simulink model "GolfSwingZVCF"  (R2024b)
settings: Solver=VariableStepAuto  StartTime=0.0  StopTime=StopTime  MaxStep=0.001  RelTol=1e-3
PreLoadFcn:
  | cd(matlabdrive);
  | cd '2DModel';
PostLoadFcn:
  | %run SCRIPT_mdlWksGenerate.m;
  | mdlWks=get_param('GolfSwingZVCF','ModelWorkspace');
  | mdlWks.DataSource = 'MAT-File';
  | mdlWks.FileName = 'ModelInputs.mat';
  | mdlWks.reload;
model workspace: external: MAT-File ModelInputsZVCF.mat (data not in the file)
undefined symbols (not defined in the file): JointTorqueHip, JointTorqueLElbow, JointTorqueLScap, JointTorqueLShoulder, JointTorqueLWrist, JointTorqueRElbow, JointTorqueRScap, JointTorqueRShoulder, JointTorqueRWrist, JointTorqueTorso, X, Y, Z
libraries: nesl_utility x286, sm_lib x176, matrix_library x11, simulink_extras x2
(part 4 of 9)

== system GolfSwingZVCF/Club/ButtGlobal ==
  Buttx : nesl_utility/PS-Simulink Converter  PhysicalDomain=network_engine_domain  SubClassName=ps_output  LeftPortType=input  RightPortType=output  PseudoPeriodic=off  Frequencies=[]  VectorFormat=1-D array  Unit=inherit  AffineConversion=off
  Butty : nesl_utility/PS-Simulink Converter  PhysicalDomain=network_engine_domain  SubClassName=ps_output  LeftPortType=input  RightPortType=output  PseudoPeriodic=off  Frequencies=[]  VectorFormat=1-D array  Unit=inherit  AffineConversion=off
  Buttz : nesl_utility/PS-Simulink Converter  PhysicalDomain=network_engine_domain  SubClassName=ps_output  LeftPortType=input  RightPortType=output  PseudoPeriodic=off  Frequencies=[]  VectorFormat=1-D array  Unit=inherit  AffineConversion=off
  Transform Sensor : sm_lib/Frames and Transforms/Transform Sensor  MeasurementFrame=World  RotationSequence=XYX  SenseAngle=off  SenseAxis=off  SenseQ=off  SenseR=off  SenseRotationSequence=off  SenseOmegaX=off  SenseOmegaY=off  SenseOmegaZ=off  SenseOmega=off  SenseQDot=off  SenseRDot=off  SenseRotationSequenceDot=off  SenseAlphaX=off  SenseAlphaY=off  SenseAlphaZ=off  SenseAlpha=off  SenseQDDot=off  SenseRDDot=off  SenseX=on  SenseY=on  SenseZ=on  SenseXYZ=off  SenseRad=off  SenseAzim=off  SenseDist=off  SenseInc=off  SenseXDot=off  SenseYDot=off  SenseZDot=off  SenseXYZDot=off  SenseRadDot=off  SenseAzimDot=off  SenseDistDot=off  SenseIncDot=off  SenseXDDot=off  SenseYDDot=off  SenseZDDot=off  SenseXYZDDot=off  SenseRadDDot=off  SenseAzimDDot=off  SenseDistDDot=off  SenseIncDDot=off
  Conn1 : PMIOPort  Side=Right
  Conn2 : PMIOPort  Port=2  Side=Left
  connections:
  Buttx/LConn1 -- Transform Sensor/RConn2
  Buttz/LConn1 -- Transform Sensor/RConn4
  Butty/LConn1 -- Transform Sensor/RConn3
  Transform Sensor/LConn1 -- Conn2/RConn1
  Transform Sensor/RConn1 -- Conn1/RConn1

== system GolfSwingZVCF/Club/CHGlobal ==
  AoA Calculation : Subsystem
  CHS (m/s) : Subsystem
  CHSmph : Gain  Gain=2.23694
  CHvx : nesl_utility/PS-Simulink Converter  PhysicalDomain=network_engine_domain  SubClassName=ps_output  LeftPortType=input  RightPortType=output  PseudoPeriodic=off  Frequencies=[]  VectorFormat=1-D array  Unit=inherit  AffineConversion=off
  CHvy : nesl_utility/PS-Simulink Converter  PhysicalDomain=network_engine_domain  SubClassName=ps_output  LeftPortType=input  RightPortType=output  PseudoPeriodic=off  Frequencies=[]  VectorFormat=1-D array  Unit=inherit  AffineConversion=off
  CHvz : nesl_utility/PS-Simulink Converter  PhysicalDomain=network_engine_domain  SubClassName=ps_output  LeftPortType=input  RightPortType=output  PseudoPeriodic=off  Frequencies=[]  VectorFormat=1-D array  Unit=inherit  AffineConversion=off
  CHx : nesl_utility/PS-Simulink Converter  PhysicalDomain=network_engine_domain  SubClassName=ps_output  LeftPortType=input  RightPortType=output  PseudoPeriodic=off  Frequencies=[]  VectorFormat=1-D array  Unit=inherit  AffineConversion=off
  CHy : nesl_utility/PS-Simulink Converter  PhysicalDomain=network_engine_domain  SubClassName=ps_output  LeftPortType=input  RightPortType=output  PseudoPeriodic=off  Frequencies=[]  VectorFormat=1-D array  Unit=inherit  AffineConversion=off
  CHz : nesl_utility/PS-Simulink Converter  PhysicalDomain=network_engine_domain  SubClassName=ps_output  LeftPortType=input  RightPortType=output  PseudoPeriodic=off  Frequencies=[]  VectorFormat=1-D array  Unit=inherit  AffineConversion=off
  ClubheadPathUnitVector : Mux  Inputs=3
  Filtering Block : Subsystem  Commented=on
  Path Calculation : Subsystem
  Transform Sensor : sm_lib/Frames and Transforms/Transform Sensor  MeasurementFrame=World  RotationSequence=XYX  SenseAngle=off  SenseAxis=off  SenseQ=off  SenseR=off  SenseRotationSequence=off  SenseOmegaX=off  SenseOmegaY=off  SenseOmegaZ=off  SenseOmega=off  SenseQDot=off  SenseRDot=off  SenseRotationSequenceDot=off  SenseAlphaX=off  SenseAlphaY=off  SenseAlphaZ=off  SenseAlpha=off  SenseQDDot=off  SenseRDDot=off  SenseX=on  SenseY=on  SenseZ=on  SenseXYZ=off  SenseRad=off  SenseAzim=off  SenseDist=off  SenseInc=off  SenseXDot=on  SenseYDot=on  SenseZDot=on  SenseXYZDot=off  SenseRadDot=off  SenseAzimDot=off  SenseDistDot=off  SenseIncDot=off  SenseXDDot=off  SenseYDDot=off  SenseZDDot=off  SenseXYZDDot=off  SenseRadDDot=off  SenseAzimDDot=off  SenseDistDDot=off  SenseIncDDot=off
  UnitVectorX : Product  Inputs=*/
  UnitVectorY : Product  Inputs=*/
  UnitVectorZ : Product  Inputs=*/
  Clubhead : PMIOPort  Side=Right
  Global : PMIOPort  Port=2  Side=Left
  ClubPathUV : Outport
  CHSMPS : Outport  Port=2
  wires:
  CHvy/1 -> Path Calculation/1(Vy), AoA Calculation/2(Vy), UnitVectorY/1, CHS (m/s)/2(In2)  "CHvy"
  CHvx/1 -> AoA Calculation/1(Vx), Path Calculation/2(Vx), UnitVectorX/1, CHS (m/s)/1(In1)  "CHvx"
  CHvz/1 -> CHS (m/s)/3(In3), AoA Calculation/3(Vz), UnitVectorZ/1  "CHvz"
  UnitVectorZ/1 -> ClubheadPathUnitVector/3
  UnitVectorY/1 -> ClubheadPathUnitVector/2
  CHS (m/s)/1(ClubPathUV1) -> CHSMPS/1, CHSmph/1, UnitVectorZ/2, UnitVectorY/2, UnitVectorX/2  "CHSmpersec"
  UnitVectorX/1 -> ClubheadPathUnitVector/1
  ClubheadPathUnitVector/1 -> ClubPathUV/1  "ClubPathUV"
  CHSmph/1 -> Filtering Block/1(CHS (mph))  "CHS (mph)"
  connections:
  CHx/LConn1 -- Transform Sensor/RConn2
  CHz/LConn1 -- Transform Sensor/RConn4
  CHvz/LConn1 -- Transform Sensor/RConn7
  CHy/LConn1 -- Transform Sensor/RConn3
  Transform Sensor/RConn5 -- CHvx/LConn1
  CHvy/LConn1 -- Transform Sensor/RConn6
  Transform Sensor/LConn1 -- Global/RConn1
  Transform Sensor/RConn1 -- Clubhead/RConn1

== system GolfSwingZVCF/Club/Club COM Calculation ==
  Club COM : nesl_utility/PS-Simulink Converter  PhysicalDomain=network_engine_domain  SubClassName=ps_output  LeftPortType=input  RightPortType=output  PseudoPeriodic=off  Frequencies=[]  VectorFormat=1-D array  Unit=inherit  AffineConversion=off
  Club Mass : nesl_utility/PS-Simulink Converter  PhysicalDomain=network_engine_domain  SubClassName=ps_output  LeftPortType=input  RightPortType=output  PseudoPeriodic=off  Frequencies=[]  VectorFormat=1-D array  Unit=inherit  AffineConversion=off
  Inertia Sensor : sm_lib/Body Elements/Inertia Sensor  SensorExtent=BodyGroup  SpanWeldJoints=on  ExcludeGroundedBodies=off  MeasurementFrame=World  SenseMass=on  SenseCenterOfMass=on  SenseInertiaMatrix=off  SenseCenteredInertiaMatrix=off  SensePrincipalInertiaMatrix=off  SenseRotationMatrix=off  GraphicType=None  PrincipalInertiaFrameSize=20  GraphicVisPropType=SimpleVisualProperties  GraphicDiffuseColor=[0.5 0.5 0.5]  GraphicOpacity=1.0  GraphicSpecularColor=[0.5 0.5 0.5 1.0]  GraphicAmbientColor=[0.15 0.15 0.15 1.0]  GraphicEmissiveColor=[0.0 0.0 0.0 1.0]  GraphicShininess=75
  Club : PMIOPort  Side=Left
  ClubCOM : Outport
  wires:
  Club COM/1 -> ClubCOM/1  "ClubCOM"
  connections:
  Club COM/LConn1 -- Inertia Sensor/RConn2
  Inertia Sensor/LConn1 -- Club/RConn1
  Inertia Sensor/RConn1 -- Club Mass/LConn1

== system GolfSwingZVCF/Club/Clubhead Air Resistance Calculator ==
  CHSmps : Inport
  ClubPathUV : Inport  Port=2
  Add : Sum  Inputs=+++
  Air Resistance : sm_lib/Forces and Torques/External Force and Torque  EnableForceX=off  EnableForceY=off  EnableForceZ=off  EnableForce=on  ForceResolutionFrame=World  EnableTorqueX=off  EnableTorqueY=off  EnableTorqueZ=off  EnableTorque=off  TorqueResolutionFrame=AttachedFrame
  Demux : Demux  Outputs=3
  Drag Function : MATLAB Function  TreatAsAtomicUnit=on
  Math Function : Math  Operator=square
  Math Function1 : Math  Operator=square
  Math Function2 : Math  Operator=square
  Matrix Multiply : Product
  Simulink-PS Converter : nesl_utility/Simulink-PS Converter  PhysicalDomain=network_engine_domain  SubClassName=ps_input  LeftPortType=input  RightPortType=output  PseudoPeriodic=off  Frequencies=[]  NoiseDistribution=none  NoiseParameters=[]  Unit=1  AffineConversion=off  FilteringAndDerivatives=provide  SimscapeFilterOrder=1  InputFilterTimeConstant=0.001  UdotUserProvided=0
  Sqrt : Sqrt
  FDrag : PMIOPort  Side=Right
  wires:
  ClubPathUV/1 -> Matrix Multiply/2
  Matrix Multiply/1 -> Demux/1, Simulink-PS Converter/1  "FDrag"
  CHSmps/1 -> Drag Function/1(u)
  Drag Function/1(FDrag) -> Matrix Multiply/1
  Add/1 -> Sqrt/1
  Math Function2/1 -> Add/3
  Math Function/1 -> Add/1
  Math Function1/1 -> Add/2
  Demux/2 -> Math Function1/1
  Demux/1 -> Math Function/1
  Demux/3 -> Math Function2/1
  connections:
  Air Resistance/RConn1 -- FDrag/RConn1
  Simulink-PS Converter/RConn1 -- Air Resistance/LConn1

== system GolfSwingZVCF/Club/Flexible Beam Model ==
  Flexible Cylindrical Beam : sm_lib/Body Elements/Flexible Bodies/Beams/Flexible Cylindrical Beam  SectionType=Hollow  Radius=0.010  RadiusUnits=m  Thickness=0.0015  ThicknessUnits=m  Length=ShaftLength  LengthUnits=m  StiffnessAndInertiaType=CalculateFromGeometry  Density=500  DensityUnits=kg/m^3  ModuliType=YoungsPoissons  YoungsModulus=ShaftStiffness  YoungsModulusUnits=GPa  PoissonsRatio=0.33  ShearModulus=26  ShearModulusUnits=GPa  GeometricCentroid=[0 0]  GeometricCentroidUnits=m  BendingCentroid=[0 0]  BendingCentroidUnits=m  ShearCenter=[0 0]  ShearCenterUnits=m  AxialRigidity=1  AxialRigidityUnits=Pa*m^2  FlexuralRigidity=[1 1]  FlexuralRigidityUnits=Pa*m^4  CrossFlexuralRigidity=0  CrossFlexuralRigidityUnits=Pa*m^4  TorsionalRigidity=1  TorsionalRigidityUnits=Pa*m^4  CenterOfMass=[0 0]  CenterOfMassUnits=m  MassPerUnitLength=1  MassPerUnitLengthUnits=kg/m  MassMomentOfInertiaDensity=[1 1]  MassMomentOfInertiaDensityUnits=kg*m  MassProductOfInertiaDensity=0  MassProductOfInertiaDensityUnits=kg*m  DampingType=Proportional  ProportionalDampingAlpha=0  ProportionalDampingAlphaUnits=1/s  ProportionalDampingBeta=ShaftDampening  ProportionalDampingBetaUnits=s  UniformModalDampingRatio=0.01  NumElements=1  ReductionType=None  NumRetainedModes=1  GraphicType=FromGeometry  GraphicVisPropType=SimpleVisualProperties  GraphicDiffuseColor=[0.5 0.5 0.5]  GraphicOpacity=1.0  GraphicSpecularColor=[0.5 0.5 0.5 1.0]  GraphicAmbientColor=[0.15 0.15 0.15 1.0]  GraphicEmissiveColor=[0.0 0.0 0.0 1.0]  GraphicShininess=75  DoExposeZminFrame=on  DoExposeZmaxFrame=on  SerializedFrames=<Frames/>
  Rigid Transform : sm_lib/Frames and Transforms/Rigid Transform  RotationMethod=RotationSequence  FollAlignAxisA=+X  BaseAlignAxisA=+Y  FollAlignAxisB=+Y  BaseAlignAxisB=+Z  RotationStandardAxis=+Z  RotationAngle=0.0  RotationAngleUnits=deg  RotationArbitraryAxis=[0 0 1]  RotationSequenceAxes=FollowerAxes  RotationSequence=XYX  RotationSequenceAngles=[0 90 0]  RotationSequenceAnglesUnits=deg  RotationMatrix=[1 0 0; 0 1 0; 0 0 1]  Quaternion=[1 0 0 0]  TranslationMethod=None  TranslationCartesianOffset=[0 0 0]  TranslationCartesianOffsetUnits=m  TranslationStandardAxis=+Z  TranslationStandardOffset=0  TranslationStandardOffsetUnits=m  TranslationROffset=0  TranslationROffsetUnits=m  TranslationThetaOffset=0  TranslationThetaOffsetUnits=deg  TranslationZOffset=0  TranslationZOffsetUnits=m
  RH Grip : PMIOPort  Side=Left
  Clubhead : PMIOPort  Port=2  Side=Right
  connections:
  Rigid Transform/RConn1 -- Flexible Cylindrical Beam/LConn1
  RH Grip/RConn1 -- Rigid Transform/LConn1
  Flexible Cylindrical Beam/RConn1 -- Clubhead/RConn1

== system GolfSwingZVCF/Club/Grip ==
  1.5 Butt : sm_lib/Body Elements/Cylindrical Solid  Commented=on  CylinderRadius=0.75  CylinderRadiusUnits=in  CylinderLength=1.5  CylinderLengthUnits=in  ExportEntireGeometry=off  InertiaType=CalculateFromGeometry  BasedOnType=Mass  Density=500  DensityUnits=kg/m^3  Mass=10  MassUnits=g  CenterOfMass=[0 0 0]  CenterOfMassUnits=m  MomentsOfInertia=[1 1 1]  MomentsOfInertiaUnits=kg*m^2  ProductsOfInertia=[0 0 0]  ProductsOfInertiaUnits=kg*m^2  GraphicType=FromGeometry  MarkerShape=Sphere  MarkerSize=10  GraphicVisPropType=SimpleVisualProperties  GraphicDiffuseColor=[0.0 0.0 0.0]  GraphicOpacity=1.0  GraphicSpecularColor=[0.5 0.5 0.5 1.0]  GraphicAmbientColor=[0.15 0.15 0.15 1.0]  GraphicEmissiveColor=[0.0 0.0 0.0 1.0]  GraphicShininess=75  DoExposeReferenceFrame=off  SerializedFrames=<Frames><Frame><Id>Frame1</Id><Value><Name>Top of Grip</Name><Origin><Source>GeometricFeature</Source><FeatureName>top curve</FeatureName></Origin><PrimaryAxis><DefinedDirection>-X</DefinedDirection><Source>ReferenceFrame</Source><SourceDirection>+Z</SourceDirection><FeatureName></FeatureName></PrimaryAxis><SecondaryAxis><DefinedDirection>+Y</DefinedDirection><Source>ReferenceFrame</Source><SourceDirection>+X</SourceDirection><FeatureName></FeatureName></SecondaryAxis></Value></Frame><Frame><Id>Frame2</Id><Value><Name>Left Hand Grip</Name><Origin><Source>GeometricFeature</Source><FeatureName>bottom curve</FeatureName></Origin><PrimaryAxis><DefinedDirection>-X</DefinedDirection><Source>ReferenceFrame</Source><SourceDirection>+Z</SourceDirection><FeatureName></FeatureName></PrimaryAxis><SecondaryAxis><DefinedDirection>+Y</DefinedDirection><Source>ReferenceFrame</Source><SourceDirection>+X</SourceDirection><FeatureName></FeatureName></SecondaryAxis></Value></Frame></Frames>
  "1.5\" Bottom" : sm_lib/Body Elements/Cylindrical Solid  CylinderRadius=0.75  CylinderRadiusUnits=in  CylinderLength=1.5  CylinderLengthUnits=in  ExportEntireGeometry=off  InertiaType=CalculateFromGeometry  BasedOnType=Mass  Density=500  DensityUnits=kg/m^3  Mass=10  MassUnits=g  CenterOfMass=[0 0 0]  CenterOfMassUnits=m  MomentsOfInertia=[1 1 1]  MomentsOfInertiaUnits=kg*m^2  ProductsOfInertia=[0 0 0]  ProductsOfInertiaUnits=kg*m^2  GraphicType=FromGeometry  MarkerShape=Sphere  MarkerSize=10  GraphicVisPropType=SimpleVisualProperties  GraphicDiffuseColor=[0.0 0.0 0.0]  GraphicOpacity=1.0  GraphicSpecularColor=[0.5 0.5 0.5 1.0]  GraphicAmbientColor=[0.15 0.15 0.15 1.0]  GraphicEmissiveColor=[0.0 0.0 0.0 1.0]  GraphicShininess=75  DoExposeReferenceFrame=off  SerializedFrames=<Frames><Frame><Id>Frame1</Id><Value><Name>Hands Midpoint</Name><Origin><Source>GeometricFeature</Source><FeatureName>top curve</FeatureName></Origin><PrimaryAxis><DefinedDirection>-X</DefinedDirection><Source>ReferenceFrame</Source><SourceDirection>+Z</SourceDirection><FeatureName></FeatureName></PrimaryAxis><SecondaryAxis><DefinedDirection>+Y</DefinedDirection><Source>ReferenceFrame</Source><SourceDirection>+X</SourceDirection><FeatureName></FeatureName></SecondaryAxis></Value></Frame><Frame><Id>Frame2</Id><Value><Name>Right Hand Grip</Name><Origin><Source>GeometricFeature</Source><FeatureName>bottom curve</FeatureName></Origin><PrimaryAxis><DefinedDirection>-X</DefinedDirection><Source>ReferenceFrame</Source><SourceDirection>+Z</SourceDirection><FeatureName></FeatureName></PrimaryAxis><SecondaryAxis><DefinedDirection>+Y</DefinedDirection><Source>ReferenceFrame</Source><SourceDirection>+X</SourceDirection><FeatureName></FeatureName></SecondaryAxis></Value></Frame></Frames>
  "1.5\" Top" : sm_lib/Body Elements/Cylindrical Solid  CylinderRadius=0.75  CylinderRadiusUnits=in  CylinderLength=1.5  CylinderLengthUnits=in  ExportEntireGeometry=off  InertiaType=CalculateFromGeometry  BasedOnType=Mass  Density=500  DensityUnits=kg/m^3  Mass=10  MassUnits=g  CenterOfMass=[0 0 0]  CenterOfMassUnits=m  MomentsOfInertia=[1 1 1]  MomentsOfInertiaUnits=kg*m^2  ProductsOfInertia=[0 0 0]  ProductsOfInertiaUnits=kg*m^2  GraphicType=FromGeometry  MarkerShape=Sphere  MarkerSize=10  GraphicVisPropType=SimpleVisualProperties  GraphicDiffuseColor=[0.0 0.0 0.0]  GraphicOpacity=1.0  GraphicSpecularColor=[0.5 0.5 0.5 1.0]  GraphicAmbientColor=[0.15 0.15 0.15 1.0]  GraphicEmissiveColor=[0.0 0.0 0.0 1.0]  GraphicShininess=75  DoExposeReferenceFrame=off  SerializedFrames=<Frames><Frame><Id>Frame1</Id><Value><Name>Left Hand Grip</Name><Origin><Source>GeometricFeature</Source><FeatureName>top curve</FeatureName></Origin><PrimaryAxis><DefinedDirection>-X</DefinedDirection><Source>ReferenceFrame</Source><SourceDirection>+Z</SourceDirection><FeatureName></FeatureName></PrimaryAxis><SecondaryAxis><DefinedDirection>+Y</DefinedDirection><Source>ReferenceFrame</Source><SourceDirection>+X</SourceDirection><FeatureName></FeatureName></SecondaryAxis></Value></Frame><Frame><Id>Frame2</Id><Value><Name>Hands Midpoint</Name><Origin><Source>GeometricFeature</Source><FeatureName>bottom curve</FeatureName></Origin><PrimaryAxis><DefinedDirection>-X</DefinedDirection><Source>ReferenceFrame</Source><SourceDirection>+Z</SourceDirection><FeatureName></FeatureName></PrimaryAxis><SecondaryAxis><DefinedDirection>+Y</DefinedDirection><Source>ReferenceFrame</Source><SourceDirection>+X</SourceDirection><FeatureName></FeatureName></SecondaryAxis></Value></Frame></Frames>
  "1.75\" Bottom" : sm_lib/Body Elements/Cylindrical Solid  Commented=on  CylinderRadius=0.75  CylinderRadiusUnits=in  CylinderLength=1.75  CylinderLengthUnits=in  ExportEntireGeometry=off  InertiaType=CalculateFromGeometry  BasedOnType=Mass  Density=500  DensityUnits=kg/m^3  Mass=11.66  MassUnits=g  CenterOfMass=[0 0 0]  CenterOfMassUnits=m  MomentsOfInertia=[1 1 1]  MomentsOfInertiaUnits=kg*m^2  ProductsOfInertia=[0 0 0]  ProductsOfInertiaUnits=kg*m^2  GraphicType=FromGeometry  MarkerShape=Sphere  MarkerSize=10  GraphicVisPropType=SimpleVisualProperties  GraphicDiffuseColor=[0.0 0.0 0.0]  GraphicOpacity=1.0  GraphicSpecularColor=[0.5 0.5 0.5 1.0]  GraphicAmbientColor=[0.15 0.15 0.15 1.0]  GraphicEmissiveColor=[0.0 0.0 0.0 1.0]  GraphicShininess=75  DoExposeReferenceFrame=off  SerializedFrames=<Frames><Frame><Id>Frame1</Id><Value><Name>Hands Midpoint</Name><Origin><Source>GeometricFeature</Source><FeatureName>top curve</FeatureName></Origin><PrimaryAxis><DefinedDirection>-X</DefinedDirection><Source>ReferenceFrame</Source><SourceDirection>+Z</SourceDirection><FeatureName></FeatureName></PrimaryAxis><SecondaryAxis><DefinedDirection>+Y</DefinedDirection><Source>ReferenceFrame</Source><SourceDirection>+X</SourceDirection><FeatureName></FeatureName></SecondaryAxis></Value></Frame><Frame><Id>Frame2</Id><Value><Name>Right Hand Grip</Name><Origin><Source>GeometricFeature</Source><FeatureName>bottom curve</FeatureName></Origin><PrimaryAxis><DefinedDirection>-X</DefinedDirection><Source>ReferenceFrame</Source><SourceDirection>+Z</SourceDirection><FeatureName></FeatureName></PrimaryAxis><SecondaryAxis><DefinedDirection>+Y</DefinedDirection><Source>ReferenceFrame</Source><SourceDirection>+X</SourceDirection><FeatureName></FeatureName></SecondaryAxis></Value></Frame></Frames>
  "1.75\" Top" : sm_lib/Body Elements/Cylindrical Solid  Commented=on  CylinderRadius=0.75  CylinderRadiusUnits=in  CylinderLength=1.75  CylinderLengthUnits=in  ExportEntireGeometry=off  InertiaType=CalculateFromGeometry  BasedOnType=Mass  Density=500  DensityUnits=kg/m^3  Mass=11.66  MassUnits=g  CenterOfMass=[0 0 0]  CenterOfMassUnits=m  MomentsOfInertia=[1 1 1]  MomentsOfInertiaUnits=kg*m^2  ProductsOfInertia=[0 0 0]  ProductsOfInertiaUnits=kg*m^2  GraphicType=FromGeometry  MarkerShape=Sphere  MarkerSize=10  GraphicVisPropType=SimpleVisualProperties  GraphicDiffuseColor=[0.0 0.0 0.0]  GraphicOpacity=1.0  GraphicSpecularColor=[0.5 0.5 0.5 1.0]  GraphicAmbientColor=[0.15 0.15 0.15 1.0]  GraphicEmissiveColor=[0.0 0.0 0.0 1.0]  GraphicShininess=75  DoExposeReferenceFrame=off  SerializedFrames=<Frames><Frame><Id>Frame1</Id><Value><Name>Left Hand Grip</Name><Origin><Source>GeometricFeature</Source><FeatureName>top curve</FeatureName></Origin><PrimaryAxis><DefinedDirection>-X</DefinedDirection><Source>ReferenceFrame</Source><SourceDirection>+Z</SourceDirection><FeatureName></FeatureName></PrimaryAxis><SecondaryAxis><DefinedDirection>+Y</DefinedDirection><Source>ReferenceFrame</Source><SourceDirection>+X</SourceDirection><FeatureName></FeatureName></SecondaryAxis></Value></Frame><Frame><Id>Frame2</Id><Value><Name>Hands Midpoint</Name><Origin><Source>GeometricFeature</Source><FeatureName>bottom curve</FeatureName></Origin><PrimaryAxis><DefinedDirection>-X</DefinedDirection><Source>ReferenceFrame</Source><SourceDirection>+Z</SourceDirection><FeatureName></FeatureName></PrimaryAxis><SecondaryAxis><DefinedDirection>+Y</DefinedDirection><Source>ReferenceFrame</Source><SourceDirection>+X</SourceDirection><FeatureName></FeatureName></SecondaryAxis></Value></Frame></Frames>
  "2\" Bottom" : sm_lib/Body Elements/Cylindrical Solid  Commented=on  CylinderRadius=0.75  CylinderRadiusUnits=in  CylinderLength=2  CylinderLengthUnits=in  ExportEntireGeometry=off  InertiaType=CalculateFromGeometry  BasedOnType=Mass  Density=500  DensityUnits=kg/m^3  Mass=13.33  MassUnits=g  CenterOfMass=[0 0 0]  CenterOfMassUnits=m  MomentsOfInertia=[1 1 1]  MomentsOfInertiaUnits=kg*m^2  ProductsOfInertia=[0 0 0]  ProductsOfInertiaUnits=kg*m^2  GraphicType=FromGeometry  MarkerShape=Sphere  MarkerSize=10  GraphicVisPropType=SimpleVisualProperties  GraphicDiffuseColor=[0.0 0.0 0.0]  GraphicOpacity=1.0  GraphicSpecularColor=[0.5 0.5 0.5 1.0]  GraphicAmbientColor=[0.15 0.15 0.15 1.0]  GraphicEmissiveColor=[0.0 0.0 0.0 1.0]  GraphicShininess=75  DoExposeReferenceFrame=off  SerializedFrames=<Frames><Frame><Id>Frame1</Id><Value><Name>Hands Midpoint</Name><Origin><Source>GeometricFeature</Source><FeatureName>top curve</FeatureName></Origin><PrimaryAxis><DefinedDirection>-X</DefinedDirection><Source>ReferenceFrame</Source><SourceDirection>+Z</SourceDirection><FeatureName></FeatureName></PrimaryAxis><SecondaryAxis><DefinedDirection>+Y</DefinedDirection><Source>ReferenceFrame</Source><SourceDirection>+X</SourceDirection><FeatureName></FeatureName></SecondaryAxis></Value></Frame><Frame><Id>Frame2</Id><Value><Name>Right Hand Grip</Name><Origin><Source>GeometricFeature</Source><FeatureName>bottom curve</FeatureName></Origin><PrimaryAxis><DefinedDirection>-X</DefinedDirection><Source>ReferenceFrame</Source><SourceDirection>+Z</SourceDirection><FeatureName></FeatureName></PrimaryAxis><SecondaryAxis><DefinedDirection>+Y</DefinedDirection><Source>ReferenceFrame</Source><SourceDirection>+X</SourceDirection><FeatureName></FeatureName></SecondaryAxis></Value></Frame></Frames>
  "2\" Butt" : sm_lib/Body Elements/Cylindrical Solid  Commented=on  CylinderRadius=0.75  CylinderRadiusUnits=in  CylinderLength=1  CylinderLengthUnits=in  ExportEntireGeometry=off  InertiaType=CalculateFromGeometry  BasedOnType=Mass  Density=500  DensityUnits=kg/m^3  Mass=13.333  MassUnits=g  CenterOfMass=[0 0 0]  CenterOfMassUnits=m  MomentsOfInertia=[1 1 1]  MomentsOfInertiaUnits=kg*m^2  ProductsOfInertia=[0 0 0]  ProductsOfInertiaUnits=kg*m^2  GraphicType=FromGeometry  MarkerShape=Sphere  MarkerSize=10  GraphicVisPropType=SimpleVisualProperties  GraphicDiffuseColor=[0.0 0.0 0.0]  GraphicOpacity=1.0  GraphicSpecularColor=[0.5 0.5 0.5 1.0]  GraphicAmbientColor=[0.15 0.15 0.15 1.0]  GraphicEmissiveColor=[0.0 0.0 0.0 1.0]  GraphicShininess=75  DoExposeReferenceFrame=off  SerializedFrames=<Frames><Frame><Id>Frame1</Id><Value><Name>Top of Grip</Name><Origin><Source>GeometricFeature</Source><FeatureName>top curve</FeatureName></Origin><PrimaryAxis><DefinedDirection>-X</DefinedDirection><Source>ReferenceFrame</Source><SourceDirection>+Z</SourceDirection><FeatureName></FeatureName></PrimaryAxis><SecondaryAxis><DefinedDirection>+Y</DefinedDirection><Source>ReferenceFrame</Source><SourceDirection>+X</SourceDirection><FeatureName></FeatureName></SecondaryAxis></Value></Frame><Frame><Id>Frame2</Id><Value><Name>Left Hand Grip</Name><Origin><Source>GeometricFeature</Source><FeatureName>bottom curve</FeatureName></Origin><PrimaryAxis><DefinedDirection>-X</DefinedDirection><Source>ReferenceFrame</Source><SourceDirection>+Z</SourceDirection><FeatureName></FeatureName></PrimaryAxis><SecondaryAxis><DefinedDirection>+Y</DefinedDirection><Source>ReferenceFrame</Source><SourceDirection>+X</SourceDirection><FeatureName></FeatureName></SecondaryAxis></Value></Frame></Frames>
  "2\" Top" : sm_lib/Body Elements/Cylindrical Solid  Commented=on  CylinderRadius=0.75  CylinderRadiusUnits=in  CylinderLength=2  CylinderLengthUnits=in  ExportEntireGeometry=off  InertiaType=CalculateFromGeometry  BasedOnType=Mass  Density=500  DensityUnits=kg/m^3  Mass=13.33  MassUnits=g  CenterOfMass=[0 0 0]  CenterOfMassUnits=m  MomentsOfInertia=[1 1 1]  MomentsOfInertiaUnits=kg*m^2  ProductsOfInertia=[0 0 0]  ProductsOfInertiaUnits=kg*m^2  GraphicType=FromGeometry  MarkerShape=Sphere  MarkerSize=10  GraphicVisPropType=SimpleVisualProperties  GraphicDiffuseColor=[0.0 0.0 0.0]  GraphicOpacity=1.0  GraphicSpecularColor=[0.5 0.5 0.5 1.0]  GraphicAmbientColor=[0.15 0.15 0.15 1.0]  GraphicEmissiveColor=[0.0 0.0 0.0 1.0]  GraphicShininess=75  DoExposeReferenceFrame=off  SerializedFrames=<Frames><Frame><Id>Frame1</Id><Value><Name>Left Hand Grip</Name><Origin><Source>GeometricFeature</Source><FeatureName>top curve</FeatureName></Origin><PrimaryAxis><DefinedDirection>-X</DefinedDirection><Source>ReferenceFrame</Source><SourceDirection>+Z</SourceDirection><FeatureName></FeatureName></PrimaryAxis><SecondaryAxis><DefinedDirection>+Y</DefinedDirection><Source>ReferenceFrame</Source><SourceDirection>+X</SourceDirection><FeatureName></FeatureName></SecondaryAxis></Value></Frame><Frame><Id>Frame2</Id><Value><Name>Hands Midpoint</Name><Origin><Source>GeometricFeature</Source><FeatureName>bottom curve</FeatureName></Origin><PrimaryAxis><DefinedDirection>-X</DefinedDirection><Source>ReferenceFrame</Source><SourceDirection>+Z</SourceDirection><FeatureName></FeatureName></PrimaryAxis><SecondaryAxis><DefinedDirection>+Y</DefinedDirection><Source>ReferenceFrame</Source><SourceDirection>+X</SourceDirection><FeatureName></FeatureName></SecondaryAxis></Value></Frame></Frames>
  "2.5\" Butt" : sm_lib/Body Elements/Cylindrical Solid  CylinderRadius=0.75  CylinderRadiusUnits=in  CylinderLength=2.5  CylinderLengthUnits=in  ExportEntireGeometry=off  InertiaType=CalculateFromGeometry  BasedOnType=Mass  Density=500  DensityUnits=kg/m^3  Mass=16.667  MassUnits=g  CenterOfMass=[0 0 0]  CenterOfMassUnits=m  MomentsOfInertia=[1 1 1]  MomentsOfInertiaUnits=kg*m^2  ProductsOfInertia=[0 0 0]  ProductsOfInertiaUnits=kg*m^2  GraphicType=FromGeometry  MarkerShape=Sphere  MarkerSize=10  GraphicVisPropType=SimpleVisualProperties  GraphicDiffuseColor=[0.0 0.0 0.0]  GraphicOpacity=1.0  GraphicSpecularColor=[0.5 0.5 0.5 1.0]  GraphicAmbientColor=[0.15 0.15 0.15 1.0]  GraphicEmissiveColor=[0.0 0.0 0.0 1.0]  GraphicShininess=75  DoExposeReferenceFrame=off  SerializedFrames=<Frames><Frame><Id>Frame1</Id><Value><Name>Top of Grip</Name><Origin><Source>GeometricFeature</Source><FeatureName>top curve</FeatureName></Origin><PrimaryAxis><DefinedDirection>-X</DefinedDirection><Source>ReferenceFrame</Source><SourceDirection>+Z</SourceDirection><FeatureName></FeatureName></PrimaryAxis><SecondaryAxis><DefinedDirection>+Y</DefinedDirection><Source>ReferenceFrame</Source><SourceDirection>+X</SourceDirection><FeatureName></FeatureName></SecondaryAxis></Value></Frame><Frame><Id>Frame2</Id><Value><Name>Left Hand Grip</Name><Origin><Source>GeometricFeature</Source><FeatureName>bottom curve</FeatureName></Origin><PrimaryAxis><DefinedDirection>-X</DefinedDirection><Source>ReferenceFrame</Source><SourceDirection>+Z</SourceDirection><FeatureName></FeatureName></PrimaryAxis><SecondaryAxis><DefinedDirection>+Y</DefinedDirection><Source>ReferenceFrame</Source><SourceDirection>+X</SourceDirection><FeatureName></FeatureName></SecondaryAxis></Value></Frame></Frames>
  GhostGripSegment : sm_lib/Body Elements/Cylindrical Solid  CylinderRadius=0.5  CylinderRadiusUnits=in  CylinderLength=5  CylinderLengthUnits=in  ExportEntireGeometry=off  InertiaType=CalculateFromGeometry  BasedOnType=Mass  Density=500  DensityUnits=kg/m^3  Mass=0  MassUnits=g  CenterOfMass=[0 0 0]  CenterOfMassUnits=m  MomentsOfInertia=[1 1 1]  MomentsOfInertiaUnits=kg*m^2  ProductsOfInertia=[0 0 0]  ProductsOfInertiaUnits=kg*m^2  GraphicType=FromGeometry  MarkerShape=Sphere  MarkerSize=10  GraphicVisPropType=SimpleVisualProperties  GraphicDiffuseColor=[0.0 0.0 0.0]  GraphicOpacity=1.0  GraphicSpecularColor=[0.5 0.5 0.5 1.0]  GraphicAmbientColor=[0.15 0.15 0.15 1.0]  GraphicEmissiveColor=[0.0 0.0 0.0 1.0]  GraphicShininess=75  DoExposeReferenceFrame=off  SerializedFrames=<Frames><Frame><Id>Frame1</Id><Value><Name>Right Hand</Name><Origin><Source>GeometricFeature</Source><FeatureName>top curve</FeatureName></Origin><PrimaryAxis><DefinedDirection>-X</DefinedDirection><Source>ReferenceFrame</Source><SourceDirection>+Z</SourceDirection><FeatureName></FeatureName></PrimaryAxis><SecondaryAxis><DefinedDirection>+Y</DefinedDirection><Source>ReferenceFrame</Source><SourceDirection>+X</SourceDirection><FeatureName></FeatureName></SecondaryAxis></Value></Frame></Frames>
  Butt : PMIOPort  Side=Right
  MP : PMIOPort  Port=2  Side=Right
  LH : PMIOPort  Port=3  Side=Right
  RH : PMIOPort  Port=4  Side=Right
  connections:
  "1.75\" Bottom"/LConn1 -- "2\" Bottom"/LConn1 -- "2\" Top"/RConn1 -- "1.5\" Bottom"/LConn1 -- MP/RConn1 -- "1.5\" Top"/RConn1 -- "1.75\" Top"/RConn1
  "1.75\" Top"/LConn1 -- "2\" Top"/LConn1 -- "1.5\" Top"/LConn1 -- "2.5\" Butt"/RConn1 -- LH/RConn1 -- 1.5 Butt/RConn1 -- "2\" Butt"/RConn1
  "1.5\" Bottom"/RConn1 -- GhostGripSegment/LConn1 -- "1.75\" Bottom"/RConn1 -- "2\" Bottom"/RConn1 -- RH/RConn1
  Butt/RConn1 -- "2\" Butt"/LConn1 -- 1.5 Butt/LConn1 -- "2.5\" Butt"/LConn1

== system GolfSwingZVCF/Club/Impact Model ==
  CHSmps : Inport
  ClubPathUV : Inport  Port=2
  Add1 : Sum
  Golf Ball Reaction Force : MATLAB Function  TreatAsAtomicUnit=on
  Golf Ball Rxn Force : sm_lib/Forces and Torques/External Force and Torque  EnableForceX=off  EnableForceY=off  EnableForceZ=off  EnableForce=on  ForceResolutionFrame=World  EnableTorqueX=off  EnableTorqueY=off  EnableTorqueZ=off  EnableTorque=off  TorqueResolutionFrame=AttachedFrame
  Matrix Multiply : Product
  Matrix Multiply1 : Product
  Simulink-PS Converter : nesl_utility/Simulink-PS Converter  PhysicalDomain=network_engine_domain  SubClassName=ps_input  LeftPortType=input  RightPortType=output  PseudoPeriodic=off  Frequencies=[]  NoiseDistribution=none  NoiseParameters=[]  Unit=1  AffineConversion=off  FilteringAndDerivatives=provide  SimscapeFilterOrder=1  InputFilterTimeConstant=0.001  UdotUserProvided=0
  Step : Step  Time=0.24  SampleTime=0
  Step1 : Step  Time=0.2405  After=-1  SampleTime=0
  FBRxn : PMIOPort  Side=Right
  wires:
  ClubPathUV/1 -> Matrix Multiply/2
  Matrix Multiply/1 -> Simulink-PS Converter/1  "FImpact"
  CHSmps/1 -> Golf Ball Reaction Force/1(u)
  Step1/1 -> Add1/2
  Step/1 -> Add1/1
  Add1/1 -> Matrix Multiply1/1
  Golf Ball Reaction Force/1(FImpact) -> Matrix Multiply1/2
  Matrix Multiply1/1 -> Matrix Multiply/1  "FImpactMag"
  connections:
  Golf Ball Rxn Force/RConn1 -- FBRxn/RConn1
  Simulink-PS Converter/RConn1 -- Golf Ball Rxn Force/LConn1

== system GolfSwingZVCF/Club/LWGlobal ==
  Add : Sum  Inputs=+++
  LWAV : nesl_utility/PS-Simulink Converter  PhysicalDomain=network_engine_domain  SubClassName=ps_output  LeftPortType=input  RightPortType=output  PseudoPeriodic=off  Frequencies=[]  VectorFormat=1-D array  Unit=inherit  AffineConversion=off
  LWvx : nesl_utility/PS-Simulink Converter  PhysicalDomain=network_engine_domain  SubClassName=ps_output  LeftPortType=input  RightPortType=output  PseudoPeriodic=off  Frequencies=[]  VectorFormat=1-D array  Unit=inherit  AffineConversion=off
  LWvy : nesl_utility/PS-Simulink Converter  PhysicalDomain=network_engine_domain  SubClassName=ps_output  LeftPortType=input  RightPortType=output  PseudoPeriodic=off  Frequencies=[]  VectorFormat=1-D array  Unit=inherit  AffineConversion=off
  LWvz : nesl_utility/PS-Simulink Converter  PhysicalDomain=network_engine_domain  SubClassName=ps_output  LeftPortType=input  RightPortType=output  PseudoPeriodic=off  Frequencies=[]  VectorFormat=1-D array  Unit=inherit  AffineConversion=off
  LWx : nesl_utility/PS-Simulink Converter  PhysicalDomain=network_engine_domain  SubClassName=ps_output  LeftPortType=input  RightPortType=output  PseudoPeriodic=off  Frequencies=[]  VectorFormat=1-D array  Unit=inherit  AffineConversion=off
  LWy : nesl_utility/PS-Simulink Converter  PhysicalDomain=network_engine_domain  SubClassName=ps_output  LeftPortType=input  RightPortType=output  PseudoPeriodic=off  Frequencies=[]  VectorFormat=1-D array  Unit=inherit  AffineConversion=off
  LWz : nesl_utility/PS-Simulink Converter  PhysicalDomain=network_engine_domain  SubClassName=ps_output  LeftPortType=input  RightPortType=output  PseudoPeriodic=off  Frequencies=[]  VectorFormat=1-D array  Unit=inherit  AffineConversion=off
  LeftHandPathUnitVector : Mux  Inputs=3
  LeftHandSpeed : Sqrt
  Math Function : Math  Operator=square
  Math Function1 : Math  Operator=square
  Math Function2 : Math  Operator=square
  Mux : Mux  Inputs=3
  Mux1 : Mux  Inputs=3
  Transform Sensor : sm_lib/Frames and Transforms/Transform Sensor  MeasurementFrame=World  RotationSequence=XYX  SenseAngle=off  SenseAxis=off  SenseQ=off  SenseR=off  SenseRotationSequence=off  SenseOmegaX=off  SenseOmegaY=off  SenseOmegaZ=off  SenseOmega=on  SenseQDot=off  SenseRDot=off  SenseRotationSequenceDot=off  SenseAlphaX=off  SenseAlphaY=off  SenseAlphaZ=off  SenseAlpha=off  SenseQDDot=off  SenseRDDot=off  SenseX=on  SenseY=on  SenseZ=on  SenseXYZ=off  SenseRad=off  SenseAzim=off  SenseDist=off  SenseInc=off  SenseXDot=on  SenseYDot=on  SenseZDot=on  SenseXYZDot=off  SenseRadDot=off  SenseAzimDot=off  SenseDistDot=off  SenseIncDot=off  SenseXDDot=off  SenseYDDot=off  SenseZDDot=off  SenseXYZDDot=off  SenseRadDDot=off  SenseAzimDDot=off  SenseDistDDot=off  SenseIncDDot=off
  UnitVectorX : Product  Inputs=*/
  UnitVectorY : Product  Inputs=*/
  UnitVectorZ : Product  Inputs=*/
  Conn1 : PMIOPort  Side=Right
  Conn2 : PMIOPort  Port=2  Side=Left
  LeftHandPathVector : Outport
  LeftHandPosition : Outport  Port=2
  LHVelocity : Outport  Port=3
  LeftWristGlobalAV : Outport  Port=4
  wires:
  LWx/1 -> Mux/1  "LWx"
  LWy/1 -> Mux/2  "LWy"
  LWz/1 -> Mux/3  "LWz"
  UnitVectorZ/1 -> LeftHandPathUnitVector/3
  UnitVectorY/1 -> LeftHandPathUnitVector/2
  LeftHandPathUnitVector/1 -> LeftHandPathVector/1  "LeftHandPathVector"
  UnitVectorX/1 -> LeftHandPathUnitVector/1
  Add/1 -> LeftHandSpeed/1
  Math Function/1 -> Add/1
  Math Function1/1 -> Add/2
  Math Function2/1 -> Add/3
  LWvy/1 -> UnitVectorY/1, Math Function1/1, Mux1/2  "LWvy"
  LeftHandSpeed/1 -> UnitVectorX/2, UnitVectorY/2, UnitVectorZ/2  "LeftHandSpeed"
  LWvz/1 -> Mux1/3, Math Function2/1, UnitVectorZ/1  "LWvz"
  LWvx/1 -> Mux1/1, UnitVectorX/1, Math Function/1  "LWvx"
  Mux/1 -> LeftHandPosition/1  "LeftHandPostion"
  Mux1/1 -> LHVelocity/1  "LeftHandVelocity"
  LWAV/1 -> LeftWristGlobalAV/1  "LeftWristGlobalAV"
  connections:
  LWx/LConn1 -- Transform Sensor/RConn3
  LWz/LConn1 -- Transform Sensor/RConn5
  LWvz/LConn1 -- Transform Sensor/RConn8
  LWy/LConn1 -- Transform Sensor/RConn4
  LWvx/LConn1 -- Transform Sensor/RConn6
  LWvy/LConn1 -- Transform Sensor/RConn7
  Transform Sensor/LConn1 -- Conn2/RConn1
  Transform Sensor/RConn1 -- Conn1/RConn1
  LWAV/LConn1 -- Transform Sensor/RConn2

== system GolfSwingZVCF/Club/Lag Angle Calculation ==
  LeftElbowGlobalPosition : Inport
  RightWristGlobalPosition : Inport  Port=2
  LeftWristGlobalPosition : Inport  Port=3
  Add : Sum  Inputs=+++
  Add1 : Sum  Inputs=+++
  Demux : Demux  Outputs=3
  Demux1 : Demux  Outputs=3
  Dot Product : DotProduct  OutDataTypeStr=Inherit: Inherit via internal rule
  ForearmUVx1 : Product  Inputs=*/
  GripUV : Product  Inputs=*/
  GripVector : Sum  Inputs=+-
  GripVector1 : Sum  Inputs=+-
  Lag Angle : Trigonometry  Operator=acos
  Lag Angle Rate of Change : Derivative
  Math Function1 : Math  Operator=square
  Math Function3 : Math  Operator=square
  Vector Magnitude : Sqrt
  Vector Magnitude1 : Sqrt
  wires:
  Demux1/1 -> Add1/1
  Demux/3 -> Add/3
  Math Function1/1 -> Demux/1
  Demux/2 -> Add/2
  Demux1/2 -> Add1/2
  Demux1/3 -> Add1/3
  Vector Magnitude1/1 -> ForearmUVx1/2
  Math Function3/1 -> Demux1/1
  Lag Angle/1 -> Lag Angle Rate of Change/1  "LagAngle"
  RightWristGlobalPosition/1 -> GripVector/1
  Dot Product/1 -> Lag Angle/1
  ForearmUVx1/1 -> Dot Product/2
  LeftElbowGlobalPosition/1 -> GripVector1/1
  GripUV/1 -> Dot Product/1
  Add1/1 -> Vector Magnitude1/1
  LeftWristGlobalPosition/1 -> GripVector/2, GripVector1/2
  GripVector/1 -> Math Function3/1, ForearmUVx1/1
  Add/1 -> Vector Magnitude/1
  GripVector1/1 -> Math Function1/1, GripUV/1
  Vector Magnitude/1 -> GripUV/2
  Demux/1 -> Add/1

== system GolfSwingZVCF/Club/MidpointGlobal ==
  Add : Sum  Inputs=+++
  Hand Speed (mph) : Gain  Gain=2.23694
  MPvx : nesl_utility/PS-Simulink Converter  PhysicalDomain=network_engine_domain  SubClassName=ps_output  LeftPortType=input  RightPortType=output  PseudoPeriodic=off  Frequencies=[]  VectorFormat=1-D array  Unit=inherit  AffineConversion=off
  MPvy : nesl_utility/PS-Simulink Converter  PhysicalDomain=network_engine_domain  SubClassName=ps_output  LeftPortType=input  RightPortType=output  PseudoPeriodic=off  Frequencies=[]  VectorFormat=1-D array  Unit=inherit  AffineConversion=off
  MPvz : nesl_utility/PS-Simulink Converter  PhysicalDomain=network_engine_domain  SubClassName=ps_output  LeftPortType=input  RightPortType=output  PseudoPeriodic=off  Frequencies=[]  VectorFormat=1-D array  Unit=inherit  AffineConversion=off
  MPx : nesl_utility/PS-Simulink Converter  PhysicalDomain=network_engine_domain  SubClassName=ps_output  LeftPortType=input  RightPortType=output  PseudoPeriodic=off  Frequencies=[]  VectorFormat=1-D array  Unit=inherit  AffineConversion=off
  MPy : nesl_utility/PS-Simulink Converter  PhysicalDomain=network_engine_domain  SubClassName=ps_output  LeftPortType=input  RightPortType=output  PseudoPeriodic=off  Frequencies=[]  VectorFormat=1-D array  Unit=inherit  AffineConversion=off
  MPz : nesl_utility/PS-Simulink Converter  PhysicalDomain=network_engine_domain  SubClassName=ps_output  LeftPortType=input  RightPortType=output  PseudoPeriodic=off  Frequencies=[]  VectorFormat=1-D array  Unit=inherit  AffineConversion=off
  Math Function : Math  Operator=square
  Math Function1 : Math  Operator=square
  Math Function2 : Math  Operator=square
  MidHandPathUnitVector : Mux  Inputs=3
  MidHandSpeed : Sqrt
  MidpointAV : nesl_utility/PS-Simulink Converter  PhysicalDomain=network_engine_domain  SubClassName=ps_output  LeftPortType=input  RightPortType=output  PseudoPeriodic=off  Frequencies=[]  VectorFormat=1-D array  Unit=inherit  AffineConversion=off
  Mux : Mux  Inputs=3
  Mux1 : Mux  Inputs=3
  Transform Sensor : sm_lib/Frames and Transforms/Transform Sensor  MeasurementFrame=World  RotationSequence=XYX  SenseAngle=off  SenseAxis=off  SenseQ=off  SenseR=off  SenseRotationSequence=off  SenseOmegaX=off  SenseOmegaY=off  SenseOmegaZ=off  SenseOmega=on  SenseQDot=off  SenseRDot=off  SenseRotationSequenceDot=off  SenseAlphaX=off  SenseAlphaY=off  SenseAlphaZ=off  SenseAlpha=off  SenseQDDot=off  SenseRDDot=off  SenseX=on  SenseY=on  SenseZ=on  SenseXYZ=off  SenseRad=off  SenseAzim=off  SenseDist=off  SenseInc=off  SenseXDot=on  SenseYDot=on  SenseZDot=on  SenseXYZDot=off  SenseRadDot=off  SenseAzimDot=off  SenseDistDot=off  SenseIncDot=off  SenseXDDot=off  SenseYDDot=off  SenseZDDot=off  SenseXYZDDot=off  SenseRadDDot=off  SenseAzimDDot=off  SenseDistDDot=off  SenseIncDDot=off
  UnitVectorX : Product  Inputs=*/
  UnitVectorY : Product  Inputs=*/
  UnitVectorZ : Product  Inputs=*/
  Conn1 : PMIOPort  Side=Right
  Conn2 : PMIOPort  Port=2  Side=Left
  HandPathVector : Outport
  MidHandPosition : Outport  Port=2
  MidHandVelocity : Outport  Port=3
  wires:
  Math Function1/1 -> Add/2
  MidHandSpeed/1 -> UnitVectorZ/2, UnitVectorY/2, UnitVectorX/2, Hand Speed (mph)/1  "MidHandSpeed"
  Math Function/1 -> Add/1
  Math Function2/1 -> Add/3
  Add/1 -> MidHandSpeed/1
  UnitVectorX/1 -> MidHandPathUnitVector/1
  UnitVectorY/1 -> MidHandPathUnitVector/2
  UnitVectorZ/1 -> MidHandPathUnitVector/3
  MidHandPathUnitVector/1 -> HandPathVector/1  "MPPathVector"
  MPy/1 -> Mux/2  "MPy"
  MPz/1 -> Mux/3  "MPz"
  Mux/1 -> MidHandPosition/1  "MidHandPosition"
  MPx/1 -> Mux/1  "MPx"
  MPvy/1 -> Math Function1/1, UnitVectorY/1, Mux1/2  "MPvy"
  MPvz/1 -> Mux1/3, UnitVectorZ/1, Math Function2/1  "MPvz"
  Mux1/1 -> MidHandVelocity/1  "MidHandVelocity"
  MPvx/1 -> Mux1/1, UnitVectorX/1, Math Function/1  "MPvx"
  connections:
  MPx/LConn1 -- Transform Sensor/RConn3
  MPz/LConn1 -- Transform Sensor/RConn5
  MPvz/LConn1 -- Transform Sensor/RConn8
  MPy/LConn1 -- Transform Sensor/RConn4
  MPvx/LConn1 -- Transform Sensor/RConn6
  MPvy/LConn1 -- Transform Sensor/RConn7
  Transform Sensor/LConn1 -- Conn2/RConn1
  Transform Sensor/RConn1 -- Conn1/RConn1
  MidpointAV/LConn1 -- Transform Sensor/RConn2

== system GolfSwingZVCF/Club/Moment of Force Calculation ==
  RWTorqueGlobal : Inport
  LWTorqueGlobal : Inport  Port=2
  LWForceGlobal : Inport  Port=3
  MPForceGlobal : Inport  Port=4
  RWForceGlobal : Inport  Port=5
  LeftWristPositionGlobal : Inport  Port=6
  MidpointPositionGlobal : Inport  Port=7
  RightWristPositionGlobal : Inport  Port=8
  ClubCOMPositionGlobal : Inport  Port=9
  Convert to Local Moment : Subsystem
  Equivalent MP Couple : Subsystem
  LH MOFGlobal : matrix_library/Cross Product
  LHRVector : Sum  Inputs=+-
  MP MOF Global : matrix_library/Cross Product
  MPRVector : Sum  Inputs=+-
  RH MOFGlobal : matrix_library/Cross Product
  RHRVector : Sum  Inputs=+-
  LeftWrist : PMIOPort  Side=Left
  Midpoint : PMIOPort  Port=2  Side=Left
  RightWrist : PMIOPort  Port=3  Side=Left
  LWMOFonClub : Outport
  RWMOFonClub : Outport  Port=2
  wires:
  RHRVector/1 -> RH MOFGlobal/1
  LHRVector/1 -> LH MOFGlobal/1
  LWForceGlobal/1 -> LH MOFGlobal/2
  LeftWristPositionGlobal/1 -> LHRVector/1
  ClubCOMPositionGlobal/1 -> RHRVector/2, MPRVector/2, LHRVector/2
  MidpointPositionGlobal/1 -> MPRVector/1
  RightWristPositionGlobal/1 -> RHRVector/1
  LH MOFGlobal/1 -> Equivalent MP Couple/1(LHMOFGlobal), Convert to Local Moment/1(LWMOFGlobal), LWMOFonClub/1  "LHMOFonClubGlobal"
  MP MOF Global/1 -> Equivalent MP Couple/2(MPMOFGlobal), Convert to Local Moment/2(MPMOFGlobal)  "MPMOFonClubGlobal"
  RH MOFGlobal/1 -> RWMOFonClub/1, Convert to Local Moment/3(RWMOFGlobal), Equivalent MP Couple/3(RHMOFGlobal)  "RHMOFonClubGlobal"
  MPForceGlobal/1 -> MP MOF Global/2
  MPRVector/1 -> MP MOF Global/1
  RWForceGlobal/1 -> RH MOFGlobal/2
  LWTorqueGlobal/1 -> Equivalent MP Couple/4(LWTorqueGlobal)
  RWTorqueGlobal/1 -> Equivalent MP Couple/5(RWTorqueGlobal)
  connections:
  Convert to Local Moment/LConn1 -- LeftWrist/RConn1
  Convert to Local Moment/LConn2 -- Equivalent MP Couple/LConn1 -- Midpoint/RConn1
  Convert to Local Moment/LConn3 -- RightWrist/RConn1

== system GolfSwingZVCF/Club/RWGlobal ==
  Add : Sum  Inputs=+++
  Math Function : Math  Operator=square
  Math Function1 : Math  Operator=square
  Math Function2 : Math  Operator=square
  Mux : Mux  Inputs=3
  Mux1 : Mux  Inputs=3
  RWAV : nesl_utility/PS-Simulink Converter  PhysicalDomain=network_engine_domain  SubClassName=ps_output  LeftPortType=input  RightPortType=output  PseudoPeriodic=off  Frequencies=[]  VectorFormat=1-D array  Unit=inherit  AffineConversion=off
  RWvx : nesl_utility/PS-Simulink Converter  PhysicalDomain=network_engine_domain  SubClassName=ps_output  LeftPortType=input  RightPortType=output  PseudoPeriodic=off  Frequencies=[]  VectorFormat=1-D array  Unit=inherit  AffineConversion=off
  RWvy : nesl_utility/PS-Simulink Converter  PhysicalDomain=network_engine_domain  SubClassName=ps_output  LeftPortType=input  RightPortType=output  PseudoPeriodic=off  Frequencies=[]  VectorFormat=1-D array  Unit=inherit  AffineConversion=off
  RWvz : nesl_utility/PS-Simulink Converter  PhysicalDomain=network_engine_domain  SubClassName=ps_output  LeftPortType=input  RightPortType=output  PseudoPeriodic=off  Frequencies=[]  VectorFormat=1-D array  Unit=inherit  AffineConversion=off
  RWx : nesl_utility/PS-Simulink Converter  PhysicalDomain=network_engine_domain  SubClassName=ps_output  LeftPortType=input  RightPortType=output  PseudoPeriodic=off  Frequencies=[]  VectorFormat=1-D array  Unit=inherit  AffineConversion=off
  RWy : nesl_utility/PS-Simulink Converter  PhysicalDomain=network_engine_domain  SubClassName=ps_output  LeftPortType=input  RightPortType=output  PseudoPeriodic=off  Frequencies=[]  VectorFormat=1-D array  Unit=inherit  AffineConversion=off
  RWz : nesl_utility/PS-Simulink Converter  PhysicalDomain=network_engine_domain  SubClassName=ps_output  LeftPortType=input  RightPortType=output  PseudoPeriodic=off  Frequencies=[]  VectorFormat=1-D array  Unit=inherit  AffineConversion=off
  RightHandPathUnitVector : Mux  Inputs=3
  RightHandSpeed : Sqrt
  Transform Sensor : sm_lib/Frames and Transforms/Transform Sensor  MeasurementFrame=World  RotationSequence=XYX  SenseAngle=off  SenseAxis=off  SenseQ=off  SenseR=off  SenseRotationSequence=off  SenseOmegaX=off  SenseOmegaY=off  SenseOmegaZ=off  SenseOmega=on  SenseQDot=off  SenseRDot=off  SenseRotationSequenceDot=off  SenseAlphaX=off  SenseAlphaY=off  SenseAlphaZ=off  SenseAlpha=off  SenseQDDot=off  SenseRDDot=off  SenseX=on  SenseY=on  SenseZ=on  SenseXYZ=off  SenseRad=off  SenseAzim=off  SenseDist=off  SenseInc=off  SenseXDot=on  SenseYDot=on  SenseZDot=on  SenseXYZDot=off  SenseRadDot=off  SenseAzimDot=off  SenseDistDot=off  SenseIncDot=off  SenseXDDot=off  SenseYDDot=off  SenseZDDot=off  SenseXYZDDot=off  SenseRadDDot=off  SenseAzimDDot=off  SenseDistDDot=off  SenseIncDDot=off
  UnitVectorX : Product  Inputs=*/
  UnitVectorY : Product  Inputs=*/
  UnitVectorZ : Product  Inputs=*/
  Conn1 : PMIOPort  Side=Right
  Conn2 : PMIOPort  Port=2  Side=Left
  RightHandPathVector : Outport
  RightHandPosition : Outport  Port=2
  RHVelocity : Outport  Port=3
  RightWristGlobalAV : Outport  Port=4
  wires:
  RightHandSpeed/1 -> UnitVectorZ/2, UnitVectorY/2, UnitVectorX/2  "RightHandSpeed"
  Math Function/1 -> Add/1
  Add/1 -> RightHandSpeed/1
  Math Function2/1 -> Add/3
  Math Function1/1 -> Add/2
  UnitVectorX/1 -> RightHandPathUnitVector/1
  RightHandPathUnitVector/1 -> RightHandPathVector/1  "RightHandPathVector"
  UnitVectorZ/1 -> RightHandPathUnitVector/3
  UnitVectorY/1 -> RightHandPathUnitVector/2
  RWy/1 -> Mux/2  "RWy"
  RWz/1 -> Mux/3  "RWz"
  Mux/1 -> RightHandPosition/1  "RightHandPosition"
  RWx/1 -> Mux/1  "RWx"
  RWvz/1 -> Math Function2/1, Mux1/3, UnitVectorZ/1  "RWvz"
  RWvy/1 -> UnitVectorY/1, Math Function1/1, Mux1/2  "RWvy"
  Mux1/1 -> RHVelocity/1  "RightHandVelocity"
  RWvx/1 -> UnitVectorX/1, Mux1/1, Math Function/1  "RWvx"
  RWAV/1 -> RightWristGlobalAV/1  "RightWristGlobalAV"
  connections:
  Transform Sensor/LConn1 -- Conn2/RConn1
  Transform Sensor/RConn1 -- Conn1/RConn1
  RWx/LConn1 -- Transform Sensor/RConn3
  RWy/LConn1 -- Transform Sensor/RConn4
  RWz/LConn1 -- Transform Sensor/RConn5
  RWvx/LConn1 -- Transform Sensor/RConn6
  RWvy/LConn1 -- Transform Sensor/RConn7
  RWvz/LConn1 -- Transform Sensor/RConn8
  RWAV/LConn1 -- Transform Sensor/RConn2

== system GolfSwingZVCF/Club/Revolute Joint Shaft Models ==
  12 Segment Shaft (1 Degree Prestress) : Subsystem  Commented=on
  "12 Segment Shaft (No Prestress) " : Subsystem  Commented=on
  RH1 : PMIOPort  Side=Right
  Clubhead1 : PMIOPort  Port=2  Side=Left
  connections:
  12 Segment Shaft (1 Degree Prestress)/RConn2 -- "12 Segment Shaft (No Prestress) "/RConn2 -- Clubhead1/RConn1
  "12 Segment Shaft (No Prestress) "/RConn1 -- 12 Segment Shaft (1 Degree Prestress)/RConn1 -- RH1/RConn1
